simulink model "MatlabLogisticEquationSimulink"  (R2017b)
settings: Solver=FixedStepAuto  StartTime=0.0  StopTime=200.00  FixedStep=0.01  RelTol=1e-3
settings Model: Creator=toni  LastModifiedBy=toni

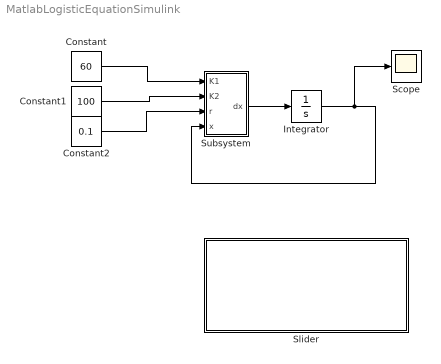
== system MatlabLogisticEquationSimulink ==
  Constant : Constant  Value=60
  Constant1 : Constant  Value=100
  Constant2 : Constant  Value=0.1
  Integrator : Integrator  InitialCondition=6.3888888888889
  Scope : Scope
  Slider : Subsystem  DialogController=hmiCreateDDGDialog  IsWebBlock=on  mask(MWDashboardBlock){webBlockId=75653ba1-0b71-4b3d-a06f-c38c6e4b8cb1, webBlockType=slider, ShowInLibBrowser=on, ShowInitialText=on, HMISrcModelName=SimulinkLogistic}
      mask prompts: webBlockId "WebBlock Id"; webBlockType "WebBlock Type"; HMISrcModelName "Source Model"
      mask help: SimulinkHMI:dialogs:SliderDialogDesc
      mask Help: helpview([docroot '/mapfiles/simulink.map'], 'hmi_slider')
      mask Display:
      | if strcmp(get_param(bdroot(gcb),'BlockDiagramType'), 'library')
      |     image([(matlabroot) '/toolbox/simulink/hmi/icons/Slider.png']);
      | end
  Subsystem : Subsystem  Description=Logistic Equation  TreatAsAtomicUnit=on
  wires:
  Subsystem/1(dx) -> Integrator/1
  Integrator/1 -> Subsystem/4("x "), Scope/1
  Constant/1 -> Subsystem/1(K1)
  Constant1/1 -> Subsystem/2(K2)
  Constant2/1 -> Subsystem/3(r)

== system MatlabLogisticEquationSimulink/Slider ==

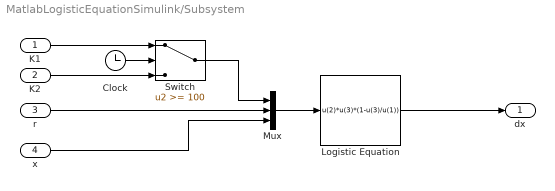
== system MatlabLogisticEquationSimulink/Subsystem ==
  K1 : Inport
  K2 : Inport  Port=2
  r : Inport  Port=3
  "x " : Inport  Port=4
  Clock : Clock
  Logistic Equation : Fcn  Expr=u(2)*u(3)*(1-u(3)/u(1))
  Mux : Mux  Inputs=3
  Switch : Switch  Threshold=100
  dx : Outport
  wires:
  Mux/1 -> Logistic Equation/1
  "x "/1 -> Mux/3
  Clock/1 -> Switch/2
  K2/1 -> Switch/3
  Switch/1 -> Mux/1
  r/1 -> Mux/2
  Logistic Equation/1 -> dx/1
  K1/1 -> Switch/1
